simulink subsystem "Reductor"  (R2023a)
settings: Solver=VariableStepAuto  StartTime=0.0  StopTime=10.0  RelTol=1e-3
model mask{J_gear=2.4, i_gear=100, vis_friction_coef_gear=0.002}
  mask prompts: J_gear "МОМЕНТ ИНЕРЦИИ"; i_gear "Передаточное число"; vis_friction_coef_gear "Коэфф. трения"
settings Model: Creator=desire  LastModifiedBy=user

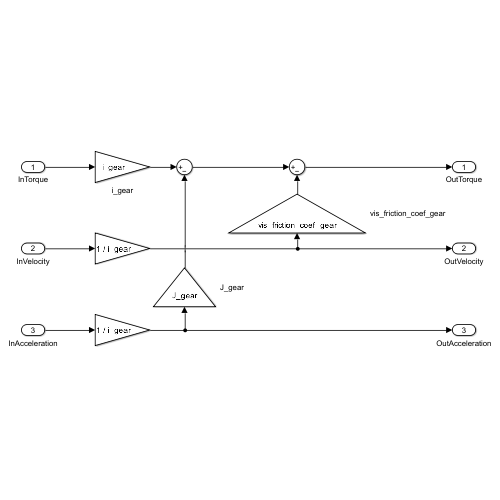
[thumbnail: Simulink's stored preview of the top-level diagram]
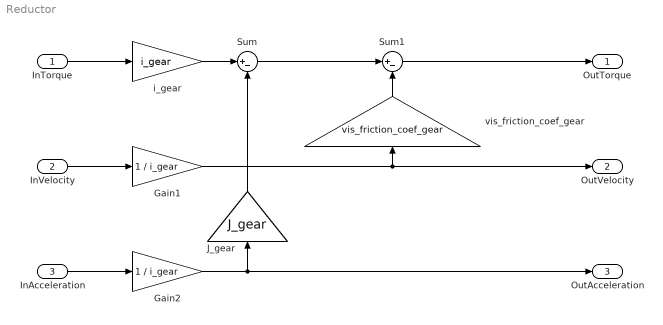
== system Reductor ==
  InTorque : Inport
  InVelocity : Inport  Port=2
  InAcceleration : Inport  Port=3
  Gain1 : Gain  Gain=1 / i_gear
  Gain2 : Gain  Gain=1 / i_gear
  J_gear : Gain  Gain=J_gear
  Sum : Sum  Inputs=|+-
  Sum1 : Sum  Inputs=|+-
  i_gear : Gain  Gain=i_gear
  vis_friction_coef_gear : Gain  Gain=vis_friction_coef_gear
  OutTorque : Outport
  OutVelocity : Outport  Port=2
  OutAcceleration : Outport  Port=3
  wires:
  Sum1/1 -> OutTorque/1
  i_gear/1 -> Sum/1
  J_gear/1 -> Sum/2
  InTorque/1 -> i_gear/1
  vis_friction_coef_gear/1 -> Sum1/2
  InAcceleration/1 -> Gain2/1
  Sum/1 -> Sum1/1
  Gain2/1 -> OutAcceleration/1, J_gear/1
  InVelocity/1 -> Gain1/1
  Gain1/1 -> OutVelocity/1, vis_friction_coef_gear/1
